simulink model "tb_PHcontr_V2"  (R2020a)
settings: Solver=ode45  StartTime=0.0  StopTime=20  MaxStep=1e-5  RelTol=1e-3
undefined symbols (not defined in the file): den_loop_filtZ, f_step, fdesignblkfcn, FPGA_CLK, FPGA_Ts, Fref, G_loopfilt, gcbh, IIR_C_X, IIR_C_X1, IIR_C_Y1, max_unwrap_periods, MAXPULSES, MECOS_cl_den, MECOS_MAX_PULSES, Nslits, num_loop_filtZ, PFD_CLK, PFD_noise_corrtime, PFD_Ts, phase_setpoint_degrees, PHCTRLR_CLK, PHCTRLR_Ts, PWM_CLK, TDC_cnt_per_period, Tref, unwrap_res_period_thr, unwrap_res_thr, wrap_detect_thr
libraries: xbsIndex_r4 x122, dspsigops x5, simulink x4, dspmlti4 x4, simulink_extras x2, dsparch4 x1, dspfdesign x1
(part 1 of 2)
settings Model: Creator=valbas  LastModifiedBy=valbas
settings SolverCC: AlgebraicLoopSolver=LineSearch

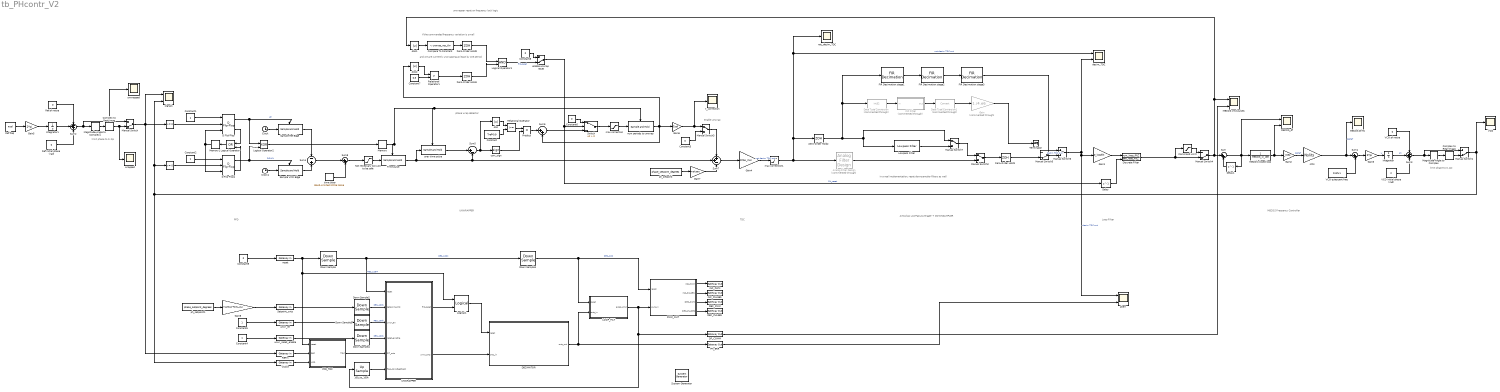
== system tb_PHcontr_V2 ==
  note: enable unwrap
  note: in a real implementation, reset downsampler filters as well
  note: if the commanded frequency variation is small
  note: unwrapper reset on frequency lock logic
  note: phase wrap detector
  note: limit phase to 0..2pi
  note: TDC
  note: AntiAlias LowPass/Averager +
      | DOWNSAMPLER
  note: Loop Filter
  note: MECOS Frequency Controller
  note: limit phase to 0..2pi
  note: PFD
  note: UNWRAPPER
  note: and we are currently unwrapping at least by one period
  " " : simulink/Logic and Bit Operations/Compare To Constant  relop=>=  const=0  OutDataTypeStr=boolean
  "  " : simulink/Logic and Bit Operations/Compare To Constant  relop=>=  const=0  OutDataTypeStr=boolean
  " System Generator" : xbsIndex_r4/ System Generator  Tag=genX  xilinxfamily=zynquplus  part=xczu7ev  speed=-2-e  package=ffvc1156  synthesis_tool=Vivado  clock_wrapper=Clock Enables  directory=./netlist  proj_type=Vivado  Synth_file=Vivado Synthesis Defaults  Impl_file=Vivado Implementation Defaults  testbench=off  simulink_period=FPGA_Ts  sysclk_period=FPGA_Ts*1e9  dcm_input_clock_period=10  incr_netlist=off  trim_vbits=Everywhere in SubSystem  dbl_ovrd=According to Block Masks  core_generation=According to Block Masks  run_coregen=off  deprecated_control=off  eval_field=0  block_type=sysgen
  100_to_100k : xbsIndex_r4/Up Sample  sample_ratio=PFD_CLK/PHCTRLR_CLK  copy_samples=on  en=off  latency=0  dbl_ovrd=off  block_type=usamp
  Abs : Abs
  Abs1 : Abs
  Abs2 : Abs
  Analog Filter Design : dsparch4/Analog Filter Design  Commented=through  method=Chebyshev II  filttype=Lowpass  N=8  Wlo=100  Whi=80  Rp=2  Rs=50
  CIC Filter : Subsystem  Commented=through  DialogController=fdesignblkfcn  InitFcn=fdesignblkfcn(gcbh, {'InitFcn'});  mask(CIC Filter){}
      mask help: Design a CIC filter
      settings: CopyFcn=fdesignblkfcn(gcbh, {'CopyFcn'});
      mask Help: helpview(mapfilelocation('dsp'), 'dspcicfilter');
      mask Display: disp('CIC')
  Clock : Clock
  Clock1 : Clock
  Command Limit : Saturate  UpperLimit=MECOS_MAX_PULSES/PHCTRLR_CLK  LowerLimit=-MECOS_MAX_PULSES/PHCTRLR_CLK
  Compare To Constant : simulink/Logic and Bit Operations/Compare To Constant  relop=<  const=unwrap_res_thr  OutDataTypeStr=boolean
  Complex to Real-Imag : ComplexToRealImag  Output=Real
  Complex to Real-Imag1 : ComplexToRealImag  Output=Real
  Constant : Constant  Value=Tref*0.9
  Constant{1..2,4..5} (4 alike) : Constant  OutDataTypeStr=boolean
  Constant3 : Constant  Value=0
  Constant6 : Constant  Value=0
  Constant7 : Constant  Value=0.5
  Constant8 : Constant  Value=0  OutDataTypeStr=boolean
  Constant9 : Constant  Value=0  OutDataTypeStr=boolean
  D Flip-Flop : simulink_extras/Flip Flops/D Flip-Flop
  D Flip-Flop1 : simulink_extras/Flip Flops/D Flip-Flop
  DECIMATOR : Subsystem
  DEC_PULSES : xbsIndex_r4/Gateway Out  inherit_from_input=on  hdl_port=on  rows=1  columns=1  UseAsDAC=off  DACChannel='1'  interface=None  automatic_assignment=on  address_offset=hex2dec('00')  intf_name=''  intf_description=''  timing_constraint=None  locs_specified=off  LOCs={}  io_standard={}  block_type=gatewayout
  DEC_PWM : xbsIndex_r4/Gateway Out  inherit_from_input=on  hdl_port=on  rows=1  columns=1  UseAsDAC=off  DACChannel='1'  interface=None  automatic_assignment=on  address_offset=hex2dec('00')  intf_name=''  intf_description=''  timing_constraint=None  locs_specified=off  LOCs={}  io_standard={}  block_type=gatewayout
  DF_COMM : xbsIndex_r4/Gateway Out  inherit_from_input=on  hdl_port=on  rows=1  columns=1  UseAsDAC=off  DACChannel='1'  interface=None  automatic_assignment=on  address_offset=hex2dec('00')  intf_name=''  intf_description=''  timing_constraint=None  locs_specified=off  LOCs={}  io_standard={}  block_type=gatewayout
  Data Type Conversion : DataTypeConversion  Commented=through  OutDataTypeStr=int32  RndMeth=Round
  Data Type Conversion1 : DataTypeConversion  Commented=through  RndMeth=Round
  Delay : Delay  DelayLength=1
  Delay1 : Delay  DelayLength=1
  Discrete Filter : DiscreteFilter  Numerator=num_loop_filtZ  Denominator=den_loop_filtZ  ExternalReset=Rising
      settings: InputPortMap=u0,r7
  Down Sample{,2..4} (4 alike) : xbsIndex_r4/Down Sample  sample_ratio=FPGA_CLK/PFD_CLK  sample_phase="Last Value of Frame  (most efficient)"  en=off  rst=off  latency=1  dbl_ovrd=off  block_type=dsamp
  Down Sample1 : xbsIndex_r4/Down Sample  sample_ratio=PFD_CLK/PHCTRLR_CLK  sample_phase="Last Value of Frame  (most efficient)"  en=off  rst=off  latency=1  dbl_ovrd=off  block_type=dsamp
  FIR Decimation stage1 : dspmlti4/FIR Decimation  FilterSource=Dialog parameters  h=Num  D=10  filtStruct=Direct form  FilterObject=FDECIM  InputProcessing=Columns as channels (frame based)  framing=Allow multirate processing  inputOffset=0  outputBufInitCond=0  roundingMode=Floor  overflowMode=off  firstCoeffDataTypeStr=Inherit: Same word length as input  firstCoeffMin=[]  firstCoeffMax=[]  firstCoeffLastDataTypeStr=Inherit: Same word length as input  outputDataTypeStr=Inherit: Same as accumulator  outputMin=[]  outputMax=[]  outputLastDataTypeStr=Inherit: Same as accumulator
  FIR Decimation stage2 : dspmlti4/FIR Decimation  FilterSource=Dialog parameters  h=Num  D=10  filtStruct=Direct form  FilterObject=FDECIM  InputProcessing=Columns as channels (frame based)  framing=Allow multirate processing  inputOffset=0  outputBufInitCond=0  roundingMode=Floor  overflowMode=off  firstCoeffDataTypeStr=Inherit: Same word length as input  firstCoeffMin=[]  firstCoeffMax=[]  firstCoeffLastDataTypeStr=Inherit: Same word length as input  outputDataTypeStr=Inherit: Same as accumulator  outputMin=[]  outputMax=[]  outputLastDataTypeStr=Inherit: Same as accumulator
  FIR Decimation stage3 : dspmlti4/FIR Decimation  FilterSource=Dialog parameters  h=Num  D=10  filtStruct=Direct form  FilterObject=FDECIM  InputProcessing=Columns as channels (frame based)  framing=Allow multirate processing  inputOffset=0  outputBufInitCond=0  roundingMode=Floor  overflowMode=off  firstCoeffDataTypeStr=Inherit: Same word length as input  firstCoeffMin=[]  firstCoeffMax=[]  firstCoeffLastDataTypeStr=Inherit: Same word length as input  outputDataTypeStr=Inherit: Same as accumulator  outputMin=[]  outputMax=[]  outputLastDataTypeStr=Inherit: Same as accumulator
  Gain : Gain  Commented=through  Gain=1./4.e6
  Gain1 : Gain  Gain=G_loopfilt
  Gain2 : Gain  Gain=f_step
  Gain3 : Gain  Gain=2*pi
  Gain4 : Gain  Gain=FPGA_CLK
  Gain5 : Gain  Gain=2*pi
  Gain6 : Gain  Gain=Tref
  Gain7 : Gain  Gain=Tref/360
  Gain8 : Gain  Gain=Tref/360*FPGA_CLK
  INC_PULSES : xbsIndex_r4/Gateway Out  inherit_from_input=on  hdl_port=on  rows=1  columns=1  UseAsDAC=off  DACChannel='1'  interface=None  automatic_assignment=on  address_offset=hex2dec('00')  intf_name=''  intf_description=''  timing_constraint=None  locs_specified=off  LOCs={}  io_standard={}  block_type=gatewayout
  INC_PWM : xbsIndex_r4/Gateway Out  inherit_from_input=on  hdl_port=on  rows=1  columns=1  UseAsDAC=off  DACChannel='1'  interface=None  automatic_assignment=on  address_offset=hex2dec('00')  intf_name=''  intf_description=''  timing_constraint=None  locs_specified=off  LOCs={}  io_standard={}  block_type=gatewayout
  Integrator : Integrator
  Integrator1 : Integrator
  LOOP_FILT : Subsystem
  Logical Operator : Logic  Operator=OR  IconShape=distinctive  AllPortsSameDT=off  OutDataTypeStr=boolean
  Logical Operator1 : Logic  IconShape=distinctive  AllPortsSameDT=off  OutDataTypeStr=boolean
  Logical Operator2 : Logic  Operator=XOR  IconShape=distinctive  AllPortsSameDT=off  OutDataTypeStr=boolean
  Logical1 : xbsIndex_r4/Logical  logical_function=OR  inputs=2  en=off  latency=0  precision=Full  arith_type=Unsigned  n_bits=16  bin_pt=0  align_bp=on  dbl_ovrd=off  block_type=logical
  Lowpass Filter : dspfdesign/Lowpass Filter  FilterType=FIR  DesignForMinimumOrder=on  FilterOrder=50  PassbandFrequency=30  StopbandFrequency=70  PassbandRipple=1  StopbandAttenuation=30  InheritSampleRate=off  SampleRate=100e3  SimulateUsing=Interpreted execution  roundingMode=Floor  coeffsDataTypeStr=fixdt(1,16)
  MECOS Df Hz : Scope
  MECOS closed loop : TransferFcn  Denominator=MECOS_cl_den
  MECOS cmd pulses : Scope  NumInputPorts=2
  MECOS_df : Scope  NumInputPorts=2
  Magnitude-Angle to Complex : MagnitudeAngleToComplex  Input=Angle  ConstantPart=1
  Magnitude-Angle to Complex1 : MagnitudeAngleToComplex  Input=Angle  ConstantPart=1
  Manual Switch{,1,4..5} (4 alike) : ManualSwitch  CurrentSetting=0
  Manual Switch{2..3,6..7} (4 alike) : ManualSwitch
  Memory : Memory
  Memory1 : Memory
  Not necessary but just to be safe : Saturate  UpperLimit=Tref  LowerLimit=-Tref
  PFD_TDC : Subsystem
  PH_ERR : xbsIndex_r4/Gateway Out  inherit_from_input=on  hdl_port=on  rows=1  columns=1  UseAsDAC=off  DACChannel='1'  interface=None  automatic_assignment=on  address_offset=hex2dec('00')  intf_name=''  intf_description=''  timing_constraint=None  locs_specified=off  LOCs={}  io_standard={}  block_type=gatewayout
  PWM_OUT : Subsystem
  Product : Product
  REFin : xbsIndex_r4/Gateway In  gui_display_data_type=Boolean  arith_type=Boolean  n_bits=16  bin_pt=14  preci_type=Single  exp_width=8  frac_width=24  rows=1  columns=1  quantization="Round  (unbiased: +/- Inf)"  overflow=Saturate  period=FPGA_Ts  UseAsADC=off  ADCChannel='1'  interface=None  automatic_assignment=on  address_offset=hex2dec('00')  intf_name=''  intf_description=''  default_value=0  timing_constraint=None  locs_specified=off  LOCs={}  io_standard={}  inherit_from_input=off  hdl_port=on  dbl_ovrd=off  block_type=gatewayin
  Ref freq : Constant  Value=Fref
  Ref initial phase (rad) : Constant  Value=0
  Ref ph noise : Constant  Value=0
  Relational Operator : RelationalOperator  OutDataTypeStr=boolean  RndMeth=Simplest
  Relational Operator1 : RelationalOperator  Operator=>  OutDataTypeStr=boolean  RndMeth=Simplest
  Sample Ref Edge : dspsigops/Sample and Hold  trig=Rising edge  initCond=0  latchinput=on
  Sample VCO Edge : dspsigops/Sample and Hold  trig=Rising edge  initCond=0  latchinput=on
  Setpoint_cnts : xbsIndex_r4/Gateway In  gui_display_data_type=Fixed-point  arith_type="Signed  (2's comp)"  n_bits=17  bin_pt=0  preci_type=Single  exp_width=8  frac_width=24  rows=1  columns=1  quantization="Round  (unbiased: +/- Inf)"  overflow=Saturate  period=FPGA_Ts  UseAsADC=off  ADCChannel='1'  interface=None  automatic_assignment=on  address_offset=hex2dec('00')  intf_name=''  intf_description=''  default_value=0  timing_constraint=None  locs_specified=off  LOCs={}  io_standard={}  inherit_from_input=off  hdl_port=on  dbl_ovrd=off  block_type=gatewayin
  Sum{,1,6,8} (4 alike) : Sum  Inputs=|++
  Sum2 : Sum  Inputs=+++
  Sum3 : Sum  Inputs=+++
  Sum4 : Sum  Inputs=-|+
  Sum5 : Sum  Inputs=|+-
  Sum7 : Sum  Inputs=++-
  Switch : Switch  Criteria=u2 > Threshold
  Terminator : Terminator
  Time pulse : dspsigops/Sample and Hold  trig=Falling edge  initCond=0  latchinput=on
  UNWRAPPER : Subsystem
  VCO : Scope
  VCO initial phase (rad) : Constant  Value=2
  VCO ph noise : Constant  Value=0
  VCO quiescent freq : Constant  Value=Fref+1
  VCOin : xbsIndex_r4/Gateway In  gui_display_data_type=Boolean  arith_type=Boolean  n_bits=16  bin_pt=14  preci_type=Single  exp_width=8  frac_width=24  rows=1  columns=1  quantization="Round  (unbiased: +/- Inf)"  overflow=Saturate  period=FPGA_Ts  UseAsADC=off  ADCChannel='1'  interface=None  automatic_assignment=on  address_offset=hex2dec('00')  intf_name=''  intf_description=''  default_value=0  timing_constraint=None  locs_specified=off  LOCs={}  io_standard={}  inherit_from_input=off  hdl_port=on  dbl_ovrd=off  block_type=gatewayin
  Zero-Order Hold1 : ZeroOrderHold  SampleTime=PHCTRLR_Ts
  Zero-Order Hold2 : ZeroOrderHold  SampleTime=PFD_Ts
  Zero-Order Hold3 : ZeroOrderHold  SampleTime=PHCTRLR_Ts
  Zero-Order Hold4 : ZeroOrderHold  SampleTime=PHCTRLR_Ts
  corr_sign : Signum
  decim_TDC : Scope  NumInputPorts=2
  enable unwrap reset : ManualSwitch  CurrentSetting=0
  max correction : Saturate  UpperLimit=max_unwrap_periods  LowerLimit=-max_unwrap_periods
  max correction1 : Saturate  UpperLimit=max_unwrap_periods*Tref*FPGA_CLK  LowerLimit=-max_unwrap_periods*Tref*FPGA_CLK
  not_decim_TDC : Scope
  num periods to unwrap : dspsigops/Sample and Hold  trig=Falling edge  initCond=0  latchinput=on
  ph_setpoint : Constant  Value=phase_setpoint_degrees
  ph_setpoint1 : Constant  Value=phase_setpoint_degrees
  pherr : Scope  NumInputPorts=2
  prev time pulse : dspsigops/Sample and Hold  trig=Falling edge  initCond=0  latchinput=on
  reset : xbsIndex_r4/Gateway In  gui_display_data_type=Boolean  arith_type=Boolean  n_bits=16  bin_pt=14  preci_type=Single  exp_width=8  frac_width=24  rows=1  columns=1  quantization="Round  (unbiased: +/- Inf)"  overflow=Saturate  period=FPGA_Ts  UseAsADC=off  ADCChannel='1'  interface=None  automatic_assignment=on  address_offset=hex2dec('00')  intf_name=''  intf_description=''  default_value=0  timing_constraint=None  locs_specified=off  LOCs={}  io_standard={}  inherit_from_input=off  hdl_port=on  dbl_ovrd=off  block_type=gatewayin
  signals : Scope  NumInputPorts=2
  slits : Gain  Gain=Nslits
  t_correction : Scope
  time jitter : simulink/Sources/Band-Limited White Noise  Cov=PFD_jitter_PSD  Ts=PFD_noise_corrtime  seed=[23341]
  unwr_en : xbsIndex_r4/Gateway In  gui_display_data_type=Boolean  arith_type=Boolean  n_bits=16  bin_pt=14  preci_type=Single  exp_width=8  frac_width=24  rows=1  columns=1  quantization="Round  (unbiased: +/- Inf)"  overflow=Saturate  period=FPGA_Ts  UseAsADC=off  ADCChannel='1'  interface=None  automatic_assignment=on  address_offset=hex2dec('00')  intf_name=''  intf_description=''  default_value=0  timing_constraint=None  locs_specified=off  LOCs={}  io_standard={}  inherit_from_input=off  hdl_port=on  dbl_ovrd=off  block_type=gatewayin
  unwr_reset_enable : xbsIndex_r4/Gateway In  gui_display_data_type=Boolean  arith_type=Boolean  n_bits=16  bin_pt=14  preci_type=Single  exp_width=8  frac_width=24  rows=1  columns=1  quantization="Round  (unbiased: +/- Inf)"  overflow=Saturate  period=FPGA_Ts  UseAsADC=off  ADCChannel='1'  interface=None  automatic_assignment=on  address_offset=hex2dec('00')  intf_name=''  intf_description=''  default_value=0  timing_constraint=None  locs_specified=off  LOCs={}  io_standard={}  inherit_from_input=off  hdl_port=on  dbl_ovrd=off  block_type=gatewayin
  unwrapped : Scope
  wrapped : Scope
  wires:
  Gain1/1 -> Discrete Filter/1
  Manual Switch6/1 -> decim_TDC/2, pherr/1, Gain1/1  "decim TDC out"
  Delay1/1 -> Sum/2
  Sum/1 -> Delay1/1, MECOS closed loop/1, MECOS_df/1
  MECOS closed loop/1 -> Gain2/1, MECOS_df/2
  slits/1 -> MECOS Df Hz/1, Sum1/1  "deltaf"
  VCO quiescent freq/1 -> Sum1/2
  Sum1/1 -> Gain3/1
  Gain3/1 -> Integrator/1  "w"
  Integrator/1 -> Sum3/2  "ph"
  Magnitude-Angle to Complex/1 -> Complex to Real-Imag1/1
  Magnitude-Angle to Complex1/1 -> Complex to Real-Imag/1
  Gain5/1 -> Integrator1/1
  Ref freq/1 -> Gain5/1
  VCO initial phase (rad)/1 -> Sum3/3
  Sum3/1 -> Manual Switch1/1, Magnitude-Angle to Complex/1
  Sum2/1 -> unwrapped/1, Manual Switch/1, Magnitude-Angle to Complex1/1
  Complex to Real-Imag/1 -> wrapped/1, Manual Switch/2
  max correction1/1 -> not_decim_TDC/1, decim_TDC/1, Zero-Order Hold2/1, Analog Filter Design/1  "not decim TDC out"
  Manual Switch/1 -> REFin/1, signals/1, " "/1
  Complex to Real-Imag1/1 -> Manual Switch1/2
  Discrete Filter/1 -> Command Limit/1, Manual Switch4/2
  Lowpass Filter/1 -> Manual Switch7/2
  Analog Filter Design/1 -> Manual Switch2/2
  Manual Switch2/1 -> Zero-Order Hold1/1
  " "/1 -> D Flip-Flop/2
  Sample Ref Edge/1 -> Sum4/1
  "  "/1 -> D Flip-Flop1/2
  Manual Switch1/1 -> VCO/1, "  "/1, signals/2, VCOin/1
  Sample VCO Edge/1 -> Sum4/2
  Clock/1 -> Sample Ref Edge/1
  Clock1/1 -> Sample VCO Edge/1
  Sum4/1 -> Sum8/1
  Logical Operator2/1 -> Memory/1
  Logical Operator/1 -> Memory1/1
  D Flip-Flop1/2 -> Logical Operator/2
  Constant2/1 -> D Flip-Flop1/1
  Memory1/1 -> D Flip-Flop1/3, D Flip-Flop/3
  D Flip-Flop/2 -> Logical Operator/1
  Constant1/1 -> D Flip-Flop/1
  D Flip-Flop/1 -> Logical Operator2/1, Sample Ref Edge/Trigger  "UP"
  D Flip-Flop1/1 -> Logical Operator2/2, Sample VCO Edge/Trigger  "DOWN"
  Sum5/1 -> Abs/1, corr_sign/1
  Constant/1 -> Relational Operator/2
  Abs/1 -> Relational Operator/1
  num periods to unwrap/1 -> Sum6/2, Abs2/1, Gain6/1
  corr_sign/1 -> Product/2
  Sum6/1 -> Switch/3
  Gain6/1 -> t_correction/1, Manual Switch3/1
  Constant3/1 -> Manual Switch3/2
  Manual Switch3/1 -> Sum7/1
  prev time pulse/1 -> Sum5/1
  Time pulse/1 -> prev time pulse/1, Sum5/2, Sum7/2
  Command Limit/1 -> Manual Switch4/1
  Not necessary but just to be safe/1 -> Time pulse/1
  Data Type Conversion/1 -> CIC Filter/1(In)
  CIC Filter/1(Out) -> Data Type Conversion1/1
  Data Type Conversion1/1 -> Gain/1
  Zero-Order Hold1/1 -> Manual Switch5/2
  Gain/1 -> Terminator/1
  Manual Switch5/1 -> Manual Switch6/2  "decim TDC out"
  FIR Decimation stage1/1 -> FIR Decimation stage2/1
  FIR Decimation stage2/1 -> FIR Decimation stage3/1
  FIR Decimation stage3/1 -> Manual Switch6/1
  Integrator1/1 -> Sum2/2
  Ref initial phase (rad)/1 -> Sum2/3
  VCO ph noise/1 -> Sum3/1
  Manual Switch7/1 -> Manual Switch2/1
  Zero-Order Hold2/1 -> FIR Decimation stage1/1, Data Type Conversion/1, Manual Switch7/1, Lowpass Filter/1
  max correction/1 -> num periods to unwrap/1
  Sum7/1 -> Gain4/1
  Gain4/1 -> max correction1/1  "not decim TDC out"
  Ref ph noise/1 -> Sum2/1
  Switch/1 -> max correction/1
  Abs1/1 -> Compare To Constant/1
  Compare To Constant/1 -> Zero-Order Hold3/1
  Relational Operator/1 -> Product/1
  Product/1 -> Sum6/1
  Memory/1 -> Time pulse/Trigger, num periods to unwrap/Trigger, prev time pulse/Trigger
  Delay/1 -> Discrete Filter/2
  Constant7/1 -> Relational Operator1/2
  Relational Operator1/1 -> Zero-Order Hold4/1
  enable unwrap reset/1 -> Delay/1, Switch/2  "filt_reset"
  Manual Switch4/1 -> Abs1/1, MECOS cmd pulses/1, Sum/1
  Zero-Order Hold4/1 -> Logical Operator1/2
  Abs2/1 -> Relational Operator1/1
  Zero-Order Hold3/1 -> Logical Operator1/1
  Constant8/1 -> enable unwrap reset/1
  ph_setpoint/1 -> Gain7/1
  Gain7/1 -> Sum7/3
  Constant6/1 -> Switch/1
  Logical Operator1/1 -> enable unwrap reset/2  "filt_reset"
  Sum8/1 -> Not necessary but just to be safe/1
  time jitter/1 -> Sum8/2
  Gain2/1 -> slits/1  "deltaf"
  ph_setpoint1/1 -> Gain8/1
  DF_COMM/1 -> MECOS cmd pulses/2
  PH_ERR/1 -> pherr/2
  unwr_reset_enable/1 -> Down Sample4/1
  PFD_TDC/1(TDC) -> UNWRAPPER/5(DT_cnts)
  Down Sample1/1 -> PWM_OUT/1(reset), LOOP_FILT/1(reset)  "RES_100"
  Down Sample4/1 -> UNWRAPPER/4(reset_enable)  "RES_100k"
  Down Sample3/1 -> UNWRAPPER/3(unwr_en)  "RES_100k"
  100_to_100k/1 -> UNWRAPPER/6(freq_corr_feedback)
  Down Sample2/1 -> UNWRAPPER/2(setpoint_cnts)  "RES_100k"
  Logical1/1 -> DECIMATOR/1(reset)
  PWM_OUT/3(DEC_PWM) -> DEC_PWM/1
  VCOin/1 -> PFD_TDC/3(VCO)
  PWM_OUT/1(INC_PWM) -> INC_PWM/1
  Setpoint_cnts/1 -> Down Sample2/1
  LOOP_FILT/1(accel_cmd) -> DF_COMM/1, 100_to_100k/1, PWM_OUT/2(puls_in)
  UNWRAPPER/1(filt_reset) -> Logical1/2
  DECIMATOR/1(cnts_out) -> PH_ERR/1, LOOP_FILT/2(cnts_in)
  PWM_OUT/2(INC_PULSES) -> INC_PULSES/1
  PWM_OUT/4(DEC_PULSES) -> DEC_PULSES/1
  Down Sample/1 -> Down Sample1/1, UNWRAPPER/1(reset)  "RES_100k"
  reset/1 -> PFD_TDC/1(reset), Logical1/1, Down Sample/1  "RES_125M"
  UNWRAPPER/2(unwr_cnts) -> DECIMATOR/2(cnts_in)
  unwr_en/1 -> Down Sample3/1
  REFin/1 -> PFD_TDC/2(REF)
  Gain8/1 -> Setpoint_cnts/1
  Constant9/1 -> reset/1
  Constant5/1 -> unwr_en/1
  Constant4/1 -> unwr_reset_enable/1

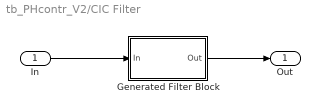
== system tb_PHcontr_V2/CIC Filter ==
  In : Inport
  Generated Filter Block : Subsystem  Tag=BlockMethodSubSystem
  Out : Outport  VectorParamsAs1DForOutWhenUnconnected=off
  wires:
  In/1 -> Generated Filter Block/1(In)
  Generated Filter Block/1(Out) -> Out/1

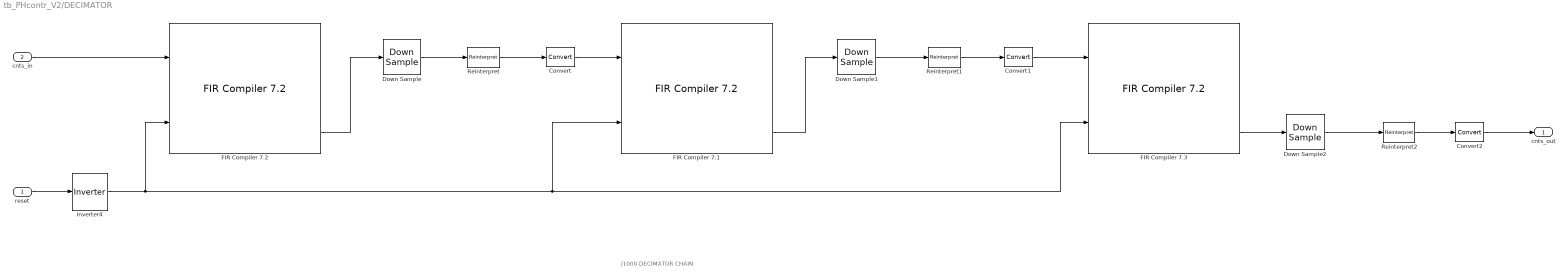
== system tb_PHcontr_V2/DECIMATOR ==
  note: /1000 DECIMATOR CHAIN
  reset : Inport  SampleTime=FPGA_Ts
  cnts_in : Inport  Port=2  SampleTime=PFD_Ts
  Convert : xbsIndex_r4/Convert  gui_display_data_type=Fixed-point  arith_type="Signed  (2's comp)"  n_bits=27  bin_pt=10  float_type=Single  exp_bits=8  fraction_bits=24  quantization="Round  (unbiased: Even Values)"  overflow=Saturate  en=off  latency=0  pipeline=off  dbl_ovrd=off  block_type=convert
  Convert1 : xbsIndex_r4/Convert  gui_display_data_type=Fixed-point  arith_type="Signed  (2's comp)"  n_bits=27  bin_pt=10  float_type=Single  exp_bits=8  fraction_bits=24  quantization="Round  (unbiased: Even Values)"  overflow=Saturate  en=off  latency=0  pipeline=off  dbl_ovrd=off  block_type=convert
  Convert2 : xbsIndex_r4/Convert  gui_display_data_type=Fixed-point  arith_type="Signed  (2's comp)"  n_bits=24  bin_pt=7  float_type=Single  exp_bits=8  fraction_bits=24  quantization="Round  (unbiased: Even Values)"  overflow=Saturate  en=off  latency=0  pipeline=off  dbl_ovrd=off  block_type=convert
  Down Sample : xbsIndex_r4/Down Sample  sample_ratio=10  sample_phase=First Value of Frame  en=off  rst=off  latency=0  dbl_ovrd=off  block_type=dsamp
  Down Sample1 : xbsIndex_r4/Down Sample  sample_ratio=10  sample_phase=First Value of Frame  en=off  rst=off  latency=0  dbl_ovrd=off  block_type=dsamp
  Down Sample2 : xbsIndex_r4/Down Sample  sample_ratio=10  sample_phase=First Value of Frame  en=off  rst=off  latency=0  dbl_ovrd=off  block_type=dsamp
  FIR Compiler 7.1 : xbsIndex_r4/FIR Compiler 7.2   coefficientvector=dectaps_int  coefficient_sets=1  coefficient_reload=off  filter_type=Single_Rate  rate_change_type=Integer  interpolation_rate=1  decimation_rate=1  zero_pack_factor=1  channel_sequence=Basic  number_channels=1  pattern_list='P4-0,P4-1,P4-2,P4-3,P4-4'  number_paths=1  ratespecification=Maximum_Possible  sampleperiod=125000  hardwareoversamplingrate=125  coefficient_sign=Signed  quantization=Integer_Coefficients  coefficient_width=18  bestprecision=off  coefficient_fractional_bits=0  coefficient_structure=Inferred  output_rounding_mode=Full_Precision  output_width=37  filter_architecture=Systolic_Multiply_Accumulate  optimization_goal=Area  optimization_list='None'  data_buffer_type=Automatic  coefficient_buffer_type=Automatic  input_buffer_type=Automatic  output_buffer_type=Automatic  preference_for_other_storage=Automatic  multi_column_support=Automatic  columnconfig='15'  inter_column_pipe_length=4  data_has_tlast=Not_Required  m_data_has_tready=off  s_data_has_fifo=off  s_data_has_tuser=Not_Required  m_data_has_tuser=Not_Required  s_config_sync_mode=On_Vector  s_config_method=Single  num_reload_slots=1  has_aclken=off  has_aresetn=on  infoeditControl=ARESETn must be asserted for a minimum of 2 cycles  reset_data_vector=on  trim_axipin_name=on  simulation_type=hybrid_sim  simulation_model=sysgen:xfirv7_2_cmodel  data_path_portlist={ 's_axis_data_tdata', 'm_axis_data_tdata' }  passband_min=0.0  passband_max=0.5  stopband_min=0.5  stopband_max=1.0  filter_selection=1  gui_behaviour='Sysgen_GUI'  data_sign=Signed  data_width=16  data_fractional_bits=0  data_tuser_width=1  wrapper_available=true  ip_wrap_arbitrary_binary_point=true  ip_name=FIR Compiler  ip_version=7.2  dsptool_ready=true  ipcore_usecache=true  ipcore_useipmodelcache=true  port_translation_map={ 'aclken' => 'en', 'aresetn' => 'rst' }  run_core_at_system_period=true  ipcore_xco_need_fpga_part=true  block_type=fir_compiler_v7_2
      settings: infoedit=Maximum Possible : Maximizes oversampling rate. Abstracted input handshake (no s_data_tvalid) and automatic rate propagation.<br>Hardware Oversampling Rate : Specifies oversampling rate relative to the input sample period. Abstracted input handshake (no s_data_tvalid) and automatic rate propagation.<br>Input/Output Sample Period : Specifies absolute oversampling rate. No input handshake abstraction (exposes s_data_tvalid) and no rate propagation.
  FIR Compiler 7.2 : xbsIndex_r4/FIR Compiler 7.2   coefficientvector=dectaps_int  coefficient_sets=1  coefficient_reload=off  filter_type=Single_Rate  rate_change_type=Integer  interpolation_rate=1  decimation_rate=1  zero_pack_factor=1  channel_sequence=Basic  number_channels=1  pattern_list='P4-0,P4-1,P4-2,P4-3,P4-4'  number_paths=1  ratespecification=Maximum_Possible  sampleperiod=125000  hardwareoversamplingrate=125  coefficient_sign=Signed  quantization=Integer_Coefficients  coefficient_width=18  bestprecision=off  coefficient_fractional_bits=0  coefficient_structure=Inferred  output_rounding_mode=Full_Precision  output_width=37  filter_architecture=Systolic_Multiply_Accumulate  optimization_goal=Area  optimization_list='None'  data_buffer_type=Automatic  coefficient_buffer_type=Automatic  input_buffer_type=Automatic  output_buffer_type=Automatic  preference_for_other_storage=Automatic  multi_column_support=Automatic  columnconfig='15'  inter_column_pipe_length=4  data_has_tlast=Not_Required  m_data_has_tready=off  s_data_has_fifo=off  s_data_has_tuser=Not_Required  m_data_has_tuser=Not_Required  s_config_sync_mode=On_Vector  s_config_method=Single  num_reload_slots=1  has_aclken=off  has_aresetn=on  infoeditControl=ARESETn must be asserted for a minimum of 2 cycles  reset_data_vector=on  trim_axipin_name=on  simulation_type=hybrid_sim  simulation_model=sysgen:xfirv7_2_cmodel  data_path_portlist={ 's_axis_data_tdata', 'm_axis_data_tdata' }  passband_min=0.0  passband_max=0.5  stopband_min=0.5  stopband_max=1.0  filter_selection=1  gui_behaviour='Sysgen_GUI'  data_sign=Signed  data_width=16  data_fractional_bits=0  data_tuser_width=1  wrapper_available=true  ip_wrap_arbitrary_binary_point=true  ip_name=FIR Compiler  ip_version=7.2  dsptool_ready=true  ipcore_usecache=true  ipcore_useipmodelcache=true  port_translation_map={ 'aclken' => 'en', 'aresetn' => 'rst' }  run_core_at_system_period=true  ipcore_xco_need_fpga_part=true  block_type=fir_compiler_v7_2
      settings: infoedit=Maximum Possible : Maximizes oversampling rate. Abstracted input handshake (no s_data_tvalid) and automatic rate propagation.<br>Hardware Oversampling Rate : Specifies oversampling rate relative to the input sample period. Abstracted input handshake (no s_data_tvalid) and automatic rate propagation.<br>Input/Output Sample Period : Specifies absolute oversampling rate. No input handshake abstraction (exposes s_data_tvalid) and no rate propagation.
  FIR Compiler 7.3 : xbsIndex_r4/FIR Compiler 7.2   coefficientvector=dectaps_int  coefficient_sets=1  coefficient_reload=off  filter_type=Single_Rate  rate_change_type=Integer  interpolation_rate=1  decimation_rate=1  zero_pack_factor=1  channel_sequence=Basic  number_channels=1  pattern_list='P4-0,P4-1,P4-2,P4-3,P4-4'  number_paths=1  ratespecification=Maximum_Possible  sampleperiod=125000  hardwareoversamplingrate=125  coefficient_sign=Signed  quantization=Integer_Coefficients  coefficient_width=18  bestprecision=off  coefficient_fractional_bits=0  coefficient_structure=Inferred  output_rounding_mode=Full_Precision  output_width=37  filter_architecture=Systolic_Multiply_Accumulate  optimization_goal=Area  optimization_list='None'  data_buffer_type=Automatic  coefficient_buffer_type=Automatic  input_buffer_type=Automatic  output_buffer_type=Automatic  preference_for_other_storage=Automatic  multi_column_support=Automatic  columnconfig='15'  inter_column_pipe_length=4  data_has_tlast=Not_Required  m_data_has_tready=off  s_data_has_fifo=off  s_data_has_tuser=Not_Required  m_data_has_tuser=Not_Required  s_config_sync_mode=On_Vector  s_config_method=Single  num_reload_slots=1  has_aclken=off  has_aresetn=on  infoeditControl=ARESETn must be asserted for a minimum of 2 cycles  reset_data_vector=on  trim_axipin_name=on  simulation_type=hybrid_sim  simulation_model=sysgen:xfirv7_2_cmodel  data_path_portlist={ 's_axis_data_tdata', 'm_axis_data_tdata' }  passband_min=0.0  passband_max=0.5  stopband_min=0.5  stopband_max=1.0  filter_selection=1  gui_behaviour='Sysgen_GUI'  data_sign=Signed  data_width=16  data_fractional_bits=0  data_tuser_width=1  wrapper_available=true  ip_wrap_arbitrary_binary_point=true  ip_name=FIR Compiler  ip_version=7.2  dsptool_ready=true  ipcore_usecache=true  ipcore_useipmodelcache=true  port_translation_map={ 'aclken' => 'en', 'aresetn' => 'rst' }  run_core_at_system_period=true  ipcore_xco_need_fpga_part=true  block_type=fir_compiler_v7_2
      settings: infoedit=Maximum Possible : Maximizes oversampling rate. Abstracted input handshake (no s_data_tvalid) and automatic rate propagation.<br>Hardware Oversampling Rate : Specifies oversampling rate relative to the input sample period. Abstracted input handshake (no s_data_tvalid) and automatic rate propagation.<br>Input/Output Sample Period : Specifies absolute oversampling rate. No input handshake abstraction (exposes s_data_tvalid) and no rate propagation.
  Inverter4 : xbsIndex_r4/Inverter  en=off  latency=0  dbl_ovrd=off  block_type=inv
  Reinterpret : xbsIndex_r4/Reinterpret  force_arith_type=off  arith_type=Unsigned  force_bin_pt=on  bin_pt=20  block_type=reinterpret
  Reinterpret1 : xbsIndex_r4/Reinterpret  force_arith_type=off  arith_type=Unsigned  force_bin_pt=on  bin_pt=30  block_type=reinterpret
  Reinterpret2 : xbsIndex_r4/Reinterpret  force_arith_type=off  arith_type=Unsigned  force_bin_pt=on  bin_pt=30  block_type=reinterpret
  cnts_out : Outport  SampleTime=PHCTRLR_Ts
  wires:
  Inverter4/1 -> FIR Compiler 7.2/2, FIR Compiler 7.1/2, FIR Compiler 7.3/2
  Down Sample2/1 -> Reinterpret2/1
  Reinterpret2/1 -> Convert2/1
  cnts_in/1 -> FIR Compiler 7.2/1
  Convert2/1 -> cnts_out/1
  reset/1 -> Inverter4/1
  Convert/1 -> FIR Compiler 7.1/1
  Down Sample1/1 -> Reinterpret1/1
  Convert1/1 -> FIR Compiler 7.3/1
  Reinterpret1/1 -> Convert1/1
  Down Sample/1 -> Reinterpret/1
  Reinterpret/1 -> Convert/1
  FIR Compiler 7.2/3 -> Down Sample/1
  FIR Compiler 7.1/3 -> Down Sample1/1
  FIR Compiler 7.3/3 -> Down Sample2/1

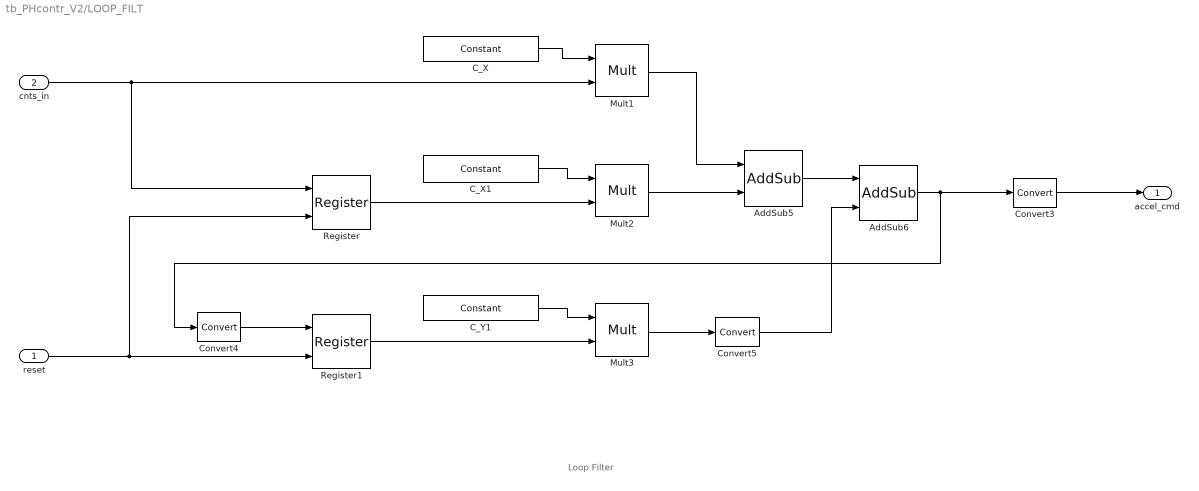
== system tb_PHcontr_V2/LOOP_FILT ==
  note: Loop Filter
  reset : Inport
  cnts_in : Inport  Port=2
  AddSub5 : xbsIndex_r4/AddSub  mode=Addition  use_carryin=off  use_carryout=off  en=off  latency=0  precision=Full  arith_type=Unsigned  n_bits=16  bin_pt=14  quantization=Truncate  overflow=Wrap  use_behavioral_HDL=off  hw_selection=Fabric  pipelined=off  dbl_ovrd=off  block_type=addsub
  AddSub6 : xbsIndex_r4/AddSub  mode=Addition  use_carryin=off  use_carryout=off  en=off  latency=0  precision=Full  arith_type=Unsigned  n_bits=16  bin_pt=14  quantization=Truncate  overflow=Wrap  use_behavioral_HDL=off  hw_selection=Fabric  pipelined=off  dbl_ovrd=off  block_type=addsub
  C_X : xbsIndex_r4/Constant  const=IIR_C_X  gui_display_data_type=Fixed-point  arith_type=Signed (2's comp)  n_bits=18  bin_pt=17  preci_type=Single  exp_width=8  frac_width=24  explicit_period=off  period=1  equ=P=C  opselect=C  inp2=PCIN>>17  opr=+  inp1=P  carry=CIN  dbl_ovrd=off  block_type=constant
  C_X1 : xbsIndex_r4/Constant  const=IIR_C_X1  gui_display_data_type=Fixed-point  arith_type=Signed (2's comp)  n_bits=18  bin_pt=17  preci_type=Single  exp_width=8  frac_width=24  explicit_period=off  period=1  equ=P=C  opselect=C  inp2=PCIN>>17  opr=+  inp1=P  carry=CIN  dbl_ovrd=off  block_type=constant
  C_Y1 : xbsIndex_r4/Constant  const=IIR_C_Y1  gui_display_data_type=Fixed-point  arith_type=Signed (2's comp)  n_bits=18  bin_pt=17  preci_type=Single  exp_width=8  frac_width=24  explicit_period=off  period=1  equ=P=C  opselect=C  inp2=PCIN>>17  opr=+  inp1=P  carry=CIN  dbl_ovrd=off  block_type=constant
  Convert3 : xbsIndex_r4/Convert  gui_display_data_type=Fixed-point  arith_type="Signed  (2's comp)"  n_bits=22  bin_pt=0  float_type=Single  exp_bits=8  fraction_bits=24  quantization="Round  (unbiased: Even Values)"  overflow=Saturate  en=off  latency=1  pipeline=off  dbl_ovrd=off  block_type=convert
  Convert4 : xbsIndex_r4/Convert  gui_display_data_type=Fixed-point  arith_type="Signed  (2's comp)"  n_bits=42  bin_pt=24  float_type=Single  exp_bits=8  fraction_bits=24  quantization="Round  (unbiased: Even Values)"  overflow=Saturate  en=off  latency=0  pipeline=off  dbl_ovrd=off  block_type=convert
  Convert5 : xbsIndex_r4/Convert  gui_display_data_type=Fixed-point  arith_type="Signed  (2's comp)"  n_bits=42  bin_pt=24  float_type=Single  exp_bits=8  fraction_bits=24  quantization="Round  (unbiased: Even Values)"  overflow=Saturate  en=off  latency=0  pipeline=off  dbl_ovrd=off  block_type=convert
  Mult1 : xbsIndex_r4/Mult  precision=Full  arith_type="Signed  (2's comp)"  n_bits=16  bin_pt=14  quantization=Truncate  overflow=Wrap  en=off  latency=0  use_behavioral_HDL=off  opt=Speed  use_embedded=on  optimum_pipeline=off  pipeline=on  dbl_ovrd=off  use_rpm=on  placement_style=Triangular  block_type=mult
  Mult2 : xbsIndex_r4/Mult  precision=Full  arith_type="Signed  (2's comp)"  n_bits=16  bin_pt=14  quantization=Truncate  overflow=Wrap  en=off  latency=0  use_behavioral_HDL=off  opt=Speed  use_embedded=on  optimum_pipeline=off  pipeline=on  dbl_ovrd=off  use_rpm=on  placement_style=Triangular  block_type=mult
  Mult3 : xbsIndex_r4/Mult  precision=Full  arith_type="Signed  (2's comp)"  n_bits=16  bin_pt=14  quantization=Truncate  overflow=Wrap  en=off  latency=0  use_behavioral_HDL=off  opt=Speed  use_embedded=on  optimum_pipeline=off  pipeline=on  dbl_ovrd=off  use_rpm=on  placement_style=Triangular  block_type=mult
  Register : xbsIndex_r4/Register  init=0  rst=on  en=off  dbl_ovrd=off  block_type=register
  Register1 : xbsIndex_r4/Register  init=0  rst=on  en=off  dbl_ovrd=off  block_type=register
  accel_cmd : Outport
  wires:
  Mult2/1 -> AddSub5/2
  Mult3/1 -> Convert5/1
  reset/1 -> Register/2, Register1/2
  Register1/1 -> Mult3/2
  AddSub5/1 -> AddSub6/1
  Mult1/1 -> AddSub5/1
  Convert5/1 -> AddSub6/2
  C_X/1 -> Mult1/1
  C_Y1/1 -> Mult3/1
  AddSub6/1 -> Convert4/1, Convert3/1
  Convert3/1 -> accel_cmd/1
  Register/1 -> Mult2/2
  cnts_in/1 -> Mult1/2, Register/1
  C_X1/1 -> Mult2/1
  Convert4/1 -> Register1/1

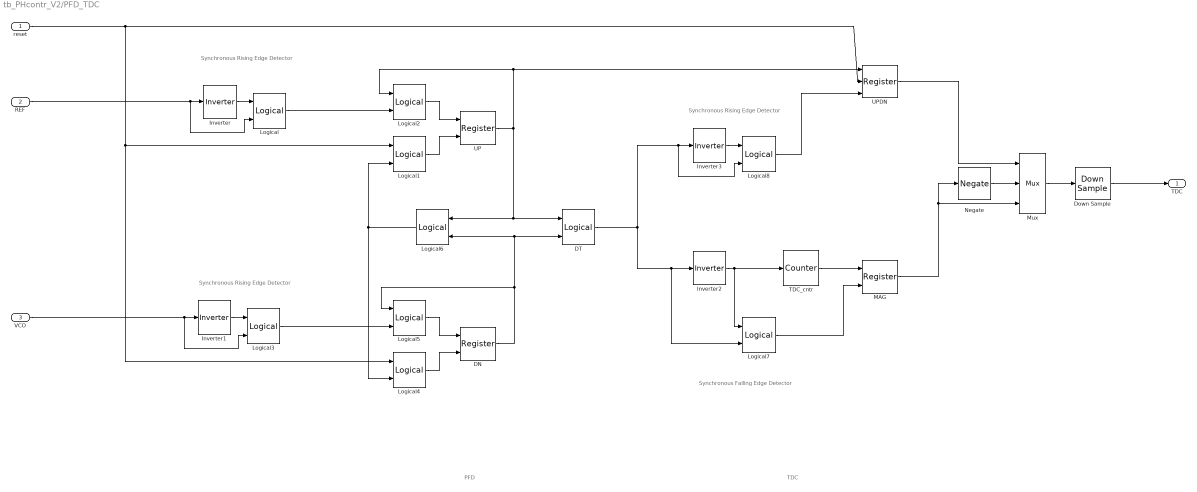
== system tb_PHcontr_V2/PFD_TDC ==
  note: Synchronous Rising Edge Detector
  note: Synchronous Rising Edge Detector
  note: Synchronous Rising Edge Detector
  note: Synchronous Falling Edge Detector
  note: PFD
  note: TDC
  reset : Inport  SampleTime=FPGA_Ts
  REF : Inport  Port=2  SampleTime=FPGA_Ts
  VCO : Inport  Port=3  SampleTime=FPGA_Ts
  DN : xbsIndex_r4/Register  init=0  rst=on  en=off  dbl_ovrd=off  block_type=register
  DT : xbsIndex_r4/Logical  logical_function=XOR  inputs=2  en=off  latency=0  precision=Full  arith_type=Unsigned  n_bits=16  bin_pt=0  align_bp=on  dbl_ovrd=off  block_type=logical
  Down Sample : xbsIndex_r4/Down Sample  sample_ratio=FPGA_CLK/PFD_CLK  sample_phase="Last Value of Frame  (most efficient)"  en=off  rst=off  latency=1  dbl_ovrd=off  block_type=dsamp
  Inverter{,1..3} (4 alike) : xbsIndex_r4/Inverter  en=off  latency=1  dbl_ovrd=off  block_type=inv
  Logical : xbsIndex_r4/Logical  logical_function=AND  inputs=2  en=off  latency=0  precision=Full  arith_type=Unsigned  n_bits=16  bin_pt=0  align_bp=on  dbl_ovrd=off  block_type=logical
  Logical{1..2,4..5} (4 alike) : xbsIndex_r4/Logical  logical_function=OR  inputs=2  en=off  latency=0  precision=Full  arith_type=Unsigned  n_bits=16  bin_pt=0  align_bp=on  dbl_ovrd=off  block_type=logical
  Logical3 : xbsIndex_r4/Logical  logical_function=AND  inputs=2  en=off  latency=0  precision=Full  arith_type=Unsigned  n_bits=16  bin_pt=0  align_bp=on  dbl_ovrd=off  block_type=logical
  Logical6 : xbsIndex_r4/Logical  logical_function=AND  inputs=2  en=off  latency=1  precision=Full  arith_type=Unsigned  n_bits=16  bin_pt=0  align_bp=on  dbl_ovrd=off  block_type=logical
  Logical7 : xbsIndex_r4/Logical  logical_function=NOR  inputs=2  en=off  latency=0  precision=Full  arith_type=Unsigned  n_bits=16  bin_pt=0  align_bp=on  dbl_ovrd=off  block_type=logical
  Logical8 : xbsIndex_r4/Logical  logical_function=AND  inputs=2  en=off  latency=0  precision=Full  arith_type=Unsigned  n_bits=16  bin_pt=0  align_bp=on  dbl_ovrd=off  block_type=logical
  MAG : xbsIndex_r4/Register  init=0  rst=off  en=on  dbl_ovrd=off  block_type=register
  Mux : xbsIndex_r4/Mux  inputs=2  en=off  latency=1  precision=Full  arith_type=Unsigned  n_bits=16  bin_pt=14  quantization=Truncate  overflow=Wrap  dbl_ovrd=off  block_type=mux
  Negate : xbsIndex_r4/Negate  precision=User Defined  arith_type="Signed  (2's comp)"  n_bits=17  bin_pt=0  quantization=Truncate  overflow=Wrap  en=off  latency=0  dbl_ovrd=off  block_type=negate
  TDC_cntr : xbsIndex_r4/Counter  cnt_type=Free Running  cnt_to=Inf  operation=Up  start_count=0  cnt_by_val=1  arith_type="Signed  (2's comp)"  n_bits=17  bin_pt=0  load_pin=off  rst=on  en=off  explicit_period=on  period=FPGA_Ts  use_behavioral_HDL=off  implementation=DSP48  dbl_ovrd=off  block_type=counter
  UP : xbsIndex_r4/Register  init=0  rst=on  en=off  dbl_ovrd=off  block_type=register
  UPDN : xbsIndex_r4/Register  init=0  rst=on  en=on  dbl_ovrd=off  block_type=register
  TDC : Outport  SampleTime=PFD_Ts
  wires:
  Inverter/1 -> Logical/1
  Logical3/1 -> Logical5/2
  VCO/1 -> Logical3/2, Inverter1/1
  reset/1 -> Logical4/1, Logical1/1, UPDN/2
  Logical5/1 -> DN/1
  Logical2/1 -> UP/1
  DN/1 -> Logical5/1, Logical6/2, DT/2
  REF/1 -> Inverter/1, Logical/2
  Inverter2/1 -> Logical7/1, TDC_cntr/1
  DT/1 -> Logical7/2, Inverter2/1, Logical8/2, Inverter3/1
  Logical4/1 -> DN/2
  MAG/1 -> Negate/1, Mux/3
  Down Sample/1 -> TDC/1
  Inverter3/1 -> Logical8/1
  Logical8/1 -> UPDN/3
  UP/1 -> Logical2/1, UPDN/1, DT/1, Logical6/1
  Logical6/1 -> Logical1/2, Logical4/2
  Logical1/1 -> UP/2
  Inverter1/1 -> Logical3/1
  Logical7/1 -> MAG/2
  UPDN/1 -> Mux/1
  Mux/1 -> Down Sample/1
  Logical/1 -> Logical2/2
  Negate/1 -> Mux/2
  TDC_cntr/1 -> MAG/1

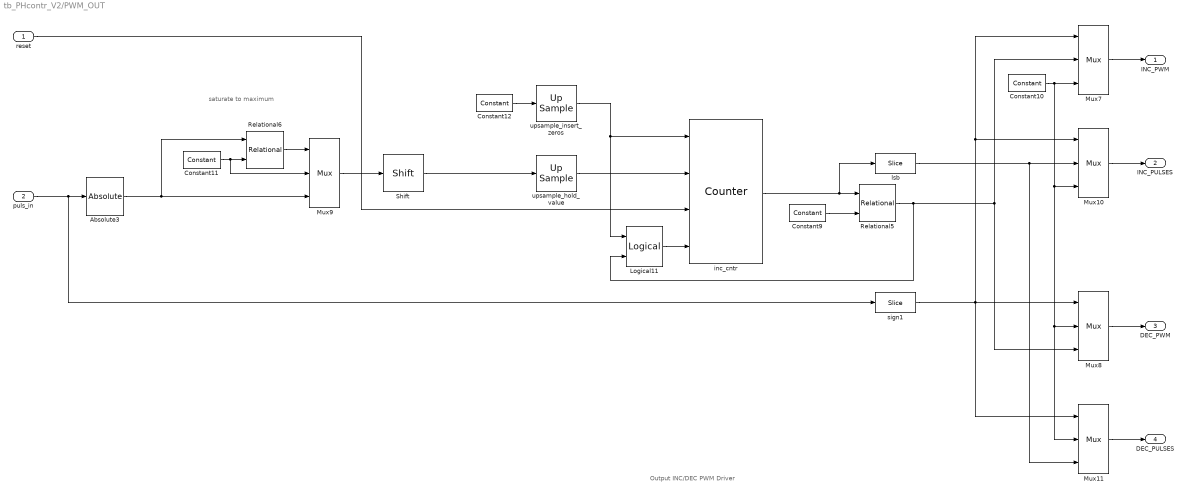
== system tb_PHcontr_V2/PWM_OUT ==
  note: saturate to maximum
  note: Output INC/DEC PWM Driver
  reset : Inport
  puls_in : Inport  Port=2
  Absolute3 : xbsIndex_r4/Absolute  precision=User Defined  arith_type="Signed  (2's comp)"  n_bits=22  bin_pt=0  quantization=Truncate  overflow=Wrap  en=off  latency=0  dbl_ovrd=off  block_type=abs
  Constant10 : xbsIndex_r4/Constant  const=0  gui_display_data_type=Boolean  arith_type=Boolean  n_bits=22  bin_pt=0  preci_type=Single  exp_width=8  frac_width=24  explicit_period=off  period=1  equ=P=C  opselect=C  inp2=PCIN>>17  opr=+  inp1=P  carry=CIN  dbl_ovrd=off  block_type=constant
  Constant11 : xbsIndex_r4/Constant  const=MAXPULSES  gui_display_data_type=Fixed-point  arith_type=Signed (2's comp)  n_bits=22  bin_pt=0  preci_type=Single  exp_width=8  frac_width=24  explicit_period=off  period=1  equ=P=C  opselect=C  inp2=PCIN>>17  opr=+  inp1=P  carry=CIN  dbl_ovrd=off  block_type=constant
  Constant12 : xbsIndex_r4/Constant  const=1  gui_display_data_type=Boolean  arith_type=Boolean  n_bits=22  bin_pt=0  preci_type=Single  exp_width=8  frac_width=24  explicit_period=on  period=PHCTRLR_Ts  equ=P=C  opselect=C  inp2=PCIN>>17  opr=+  inp1=P  carry=CIN  dbl_ovrd=off  block_type=constant
  Constant9 : xbsIndex_r4/Constant  const=0  gui_display_data_type=Fixed-point  arith_type=Signed (2's comp)  n_bits=23  bin_pt=0  preci_type=Single  exp_width=8  frac_width=24  explicit_period=off  period=1  equ=P=C  opselect=C  inp2=PCIN>>17  opr=+  inp1=P  carry=CIN  dbl_ovrd=off  block_type=constant
  Logical11 : xbsIndex_r4/Logical  logical_function=OR  inputs=2  en=off  latency=0  precision=Full  arith_type=Unsigned  n_bits=16  bin_pt=0  align_bp=on  dbl_ovrd=off  block_type=logical
  Mux{7..11} (5 alike) : xbsIndex_r4/Mux  inputs=2  en=off  latency=0  precision=Full  arith_type=Unsigned  n_bits=16  bin_pt=14  quantization=Truncate  overflow=Wrap  dbl_ovrd=off  block_type=mux
  Relational5 : xbsIndex_r4/Relational  mode=a!=b  op_type=Bool  en=off  latency=0  dbl_ovrd=off  block_type=relational
  Relational6 : xbsIndex_r4/Relational  mode=a<b  op_type=Bool  en=off  latency=0  dbl_ovrd=off  block_type=relational
  Shift : xbsIndex_r4/Shift  shift_dir=Left  shift_bits=1  en=off  latency=0  precision=User Defined  arith_type="Signed  (2's comp)"  n_bits=23  bin_pt=0  quantization=Truncate  overflow=Saturate  dbl_ovrd=off  block_type=shift
  inc_cntr : xbsIndex_r4/Counter  cnt_type=Free Running  cnt_to=0  operation=Down  start_count=0  cnt_by_val=1  arith_type="Signed  (2's comp)"  n_bits=23  bin_pt=0  load_pin=on  rst=on  en=on  explicit_period=on  period=PWM_Ts  use_behavioral_HDL=off  implementation=DSP48  dbl_ovrd=off  block_type=counter
  lsb : xbsIndex_r4/Slice  nbits=1  boolean_output=on  mode=Lower Bit Location + Width  bit1=0  base1=MSB of Input  bit0=0  base0=LSB of Input  dbl_ovrd=off  block_type=slice
  sign1 : xbsIndex_r4/Slice  nbits=1  boolean_output=on  mode=Upper Bit Location + Width  bit1=0  base1=MSB of Input  bit0=0  base0=LSB of Input  dbl_ovrd=off  block_type=slice
  upsample_hold_value : xbsIndex_r4/Up Sample  sample_ratio=PWM_CLK/PHCTRLR_CLK  copy_samples=on  en=off  latency=0  dbl_ovrd=off  block_type=usamp
  upsample_insert_zeros : xbsIndex_r4/Up Sample  sample_ratio=PWM_CLK/PHCTRLR_CLK  copy_samples=off  en=off  latency=0  dbl_ovrd=off  block_type=usamp
  INC_PWM : Outport
  INC_PULSES : Outport  Port=2
  DEC_PWM : Outport  Port=3
  DEC_PULSES : Outport  Port=4
  wires:
  Relational6/1 -> Mux9/1
  upsample_hold_value/1 -> inc_cntr/2
  reset/1 -> inc_cntr/3
  puls_in/1 -> Absolute3/1, sign1/1
  Absolute3/1 -> Relational6/1, Mux9/3
  Mux10/1 -> INC_PULSES/1
  Mux9/1 -> Shift/1
  Relational5/1 -> Logical11/2, Mux8/3, Mux7/2
  Constant12/1 -> upsample_insert_zeros/1
  lsb/1 -> Mux11/3, Mux10/2
  sign1/1 -> Mux10/1, Mux7/1, Mux11/1, Mux8/1
  upsample_insert_zeros/1 -> inc_cntr/1, Logical11/1
  Mux11/1 -> DEC_PULSES/1
  Constant11/1 -> Mux9/2, Relational6/2
  Logical11/1 -> inc_cntr/4
  Constant10/1 -> Mux11/2, Mux8/2, Mux10/3, Mux7/3
  Mux8/1 -> DEC_PWM/1
  inc_cntr/1 -> lsb/1, Relational5/1
  Shift/1 -> upsample_hold_value/1
  Constant9/1 -> Relational5/2
  Mux7/1 -> INC_PWM/1
